simulink model "Sepic_2025b"  (R2025b)
settings: Solver=VariableStepAuto  StartTime=0.0  StopTime=0.02  RelTol=1e-7  AbsTol=1e-7
undefined symbols (not defined in the file): fg_sepic, HPFenable, Ilim_sepic, Ki_sepic, Ku_sepic, R1_sepic, RL_sepic, tau_HPF_sepic, tau_PI_sepic, U2_sepic, w_Amplitude
libraries: fl_lib x14, nesl_utility x12, ee_lib x11, simulink x2, slpidlib x1
settings Model: SimulationMode=accelerator  Creator=Job  LastModifiedBy=jobme
settings SolverCC: AlgebraicLoopSolver=LineSearch  PositivePriorityOrder=on
settings DebuggingCC: UnconnectedInputMsg=warning  UnconnectedOutputMsg=warning  UnconnectedLineMsg=warning
settings HardwareCC: ProdHWDeviceType=AMD->x86-64 (Windows64)
settings ModelReferenceCC: EnableRefExpFcnMdlSchedulingChecks=on
settings SFSimCC: UsePrecompiledLibraries=Avoid  SimTargetLang=C++  GPUAcceleration=on  SimDLTargetLibrary=cudnn
settings RTWCC: GPUComputeCapability=3.5

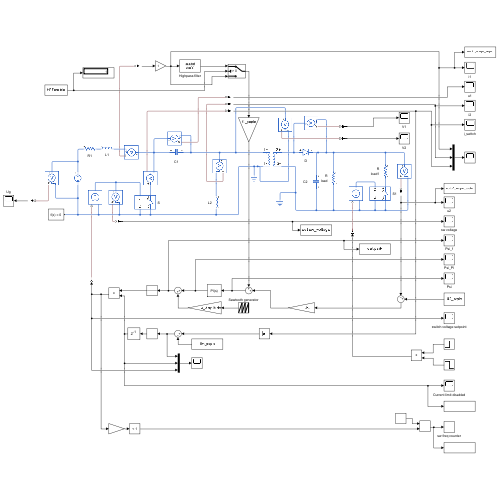
[thumbnail: Simulink's stored preview of the top-level diagram]
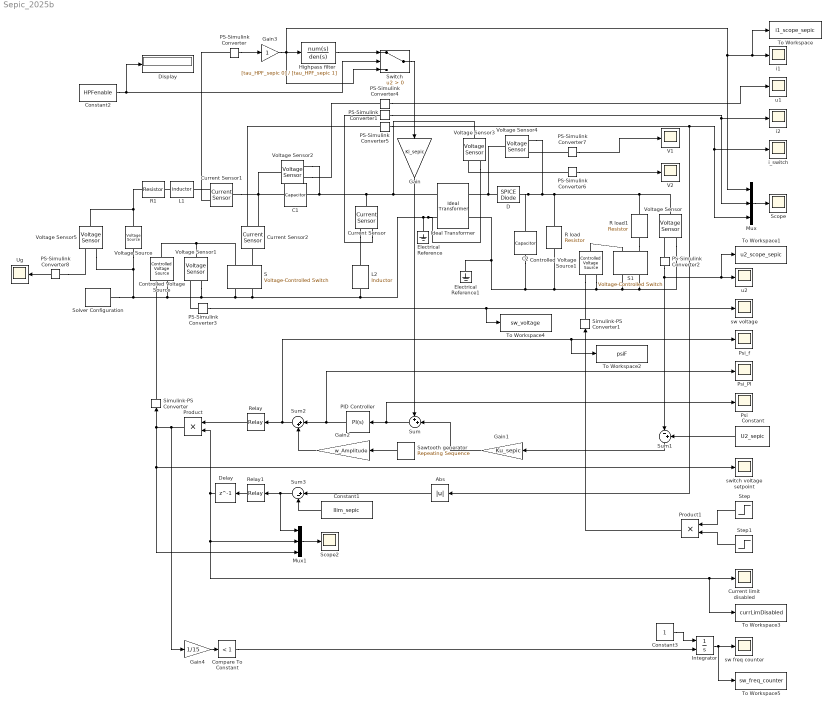
== system Sepic_2025b ==
  Abs : Abs  SaturateOnIntegerOverflow=off
  C1 : ee_lib/Passive/Capacitor  cap_option=ee.enum.passive.capacitor.capOption.const  c=C1_sepic F  Cvec=[1e-05, 1e-06] F  Vvec=[0, 10] V  CV_table_symmetry=1  f_vec=[1, 10] kHz  DFext_vec=[.8, 1.2]  enable_C_tol=0  averaging_period=0 s  C_tol=0  tol_distribution=1  nSigma=4  r=1e-6 Ohm  g=0 1/Ohm  enable_operating_limits=0  operating_limit_action=2  max_working_voltage_range=[-25, 25] V  power_rating=1 W  maxTemperature=85 degC  thermalEnable=false  thermalMass=1 J/K  i_specify=off  i_priority=None  i=0 A  i_nominal_specify=off  i_nominal_value=1  i_nominal_unit=A  v_specify=off  v_priority=None  v=0 V  v_nominal_specify=off  v_nominal_value=1  v_nominal_unit=V  vc_specify=off  vc_priority=High  vc=0 V  vc_nominal_specify=off  vc_nominal_value=1  vc_nominal_unit=V  T_specify=off  T_priority=None  T=298.15 K  T_nominal_specify=off  T_nominal_value=1  T_nominal_unit=K
  C2 : ee_lib/Passive/Capacitor  cap_option=ee.enum.passive.capacitor.capOption.const  c=C2_sepic F  Cvec=[1e-05, 1e-06] F  Vvec=[0, 10] V  CV_table_symmetry=1  f_vec=[1, 10] kHz  DFext_vec=[.8, 1.2]  enable_C_tol=0  averaging_period=0 s  C_tol=0  tol_distribution=1  nSigma=4  r=1e-6 Ohm  g=0 1/Ohm  enable_operating_limits=0  operating_limit_action=2  max_working_voltage_range=[-25, 25] V  power_rating=1 W  maxTemperature=85 degC  thermalEnable=false  thermalMass=1 J/K  i_specify=off  i_priority=None  i=0 A  i_nominal_specify=off  i_nominal_value=1  i_nominal_unit=A  v_specify=off  v_priority=None  v=0 V  v_nominal_specify=off  v_nominal_value=1  v_nominal_unit=V  vc_specify=off  vc_priority=High  vc=0 V  vc_nominal_specify=off  vc_nominal_value=1  vc_nominal_unit=V  T_specify=off  T_priority=None  T=298.15 K  T_nominal_specify=off  T_nominal_value=1  T_nominal_unit=K
  Compare To Constant : simulink/Logic and Bit Operations/Compare To Constant  relop=<  const=1  OutDataTypeStr=boolean
  Constant : Constant  Value=U2_sepic
  Constant1 : Constant  Value=Ilim_sepic
  Constant2 : Constant  Value=HPFenable
  Constant3 : Constant
  Controlled Voltage Source : fl_lib/Electrical/Electrical Sources/Controlled Voltage Source
  Controlled Voltage Source1 : fl_lib/Electrical/Electrical Sources/Controlled Voltage Source
  Current Sensor : fl_lib/Electrical/Electrical Sensors/Current Sensor
  Current Sensor1 : fl_lib/Electrical/Electrical Sensors/Current Sensor
  Current Sensor2 : fl_lib/Electrical/Electrical Sensors/Current Sensor
  Current limit disabled : Scope
      settings: ActiveDisplayYMinimum=-0.125  ActiveDisplayYMaximum=1.125  DataLoggingVariableName=currLimDisabled  DataLoggingSaveFormat=Array
  D : ee_lib/Additional Components/SPICE Semiconductors/SPICE Diode  AREA=1.0 m^2  SCALE=1  IS=1e-14 A/m^2  IKF=Inf A/m^2  ISR=0 A/m^2  N=1  NR=2  M=0.5  VJ=1 V  RS=0.01 m^2*Ohm  C_param=1  CJO=0 F/m^2  FC=0.5  TT=0 s  IC_given=1  V0=0 V  RevBrk=1  BV=Inf V  IBV=1e-3 A/m^2  IBVL=0 A/m^2  NBV=1  NBVL=1  T_param=1  XTI=3.0  EG=1.11 eV  TIKF=0 1/K  TRS1=0 1/K  TRS2=0 1/K^2  TBV1=0 1/K  TBV2=0 1/K^2  TFIXED=300.15 K  TMEAS=300.15 K  TOFFSET=0 K
      settings: InternalSimscapePortConfiguration="{\"Bottom\":[],\"Left\":[{\"id\":\"p\",\"label\":\"+\",\"type\":\"foundation.electrical.electrical\"}],\"Right\":[{\"id\":\"n\",\"label\":\"-\",\"type\":\"foundation.electrical.electrical\"}],\"Top\":[]}"
  Delay : Delay  DelayLength=1
  Display : Display
  Electrical Reference : fl_lib/Electrical/Electrical Elements/Electrical Reference
  Electrical Reference1 : fl_lib/Electrical/Electrical Elements/Electrical Reference
  Gain : Gain  Gain=Ki_sepic
  Gain1 : Gain  Gain=Ku_sepic
  Gain2 : Gain  Gain=w_Amplitude
  Gain3 : Gain
  Gain4 : Gain  Gain=1/15  OutDataTypeStr=uint8
  Highpass filter : TransferFcn  Numerator=[tau_HPF_sepic 0]  Denominator=[tau_HPF_sepic 1]
  Ideal Transformer : fl_lib/Electrical/Electrical Elements/Ideal Transformer  n=n_sepic  i1_specify=off  i1_priority=None  i1=0 A  i1_nominal_specify=off  i1_nominal_value=1  i1_nominal_unit=A  v1_specify=off  v1_priority=None  v1=0 V  v1_nominal_specify=off  v1_nominal_value=1  v1_nominal_unit=V  i2_specify=off  i2_priority=None  i2=0 A  i2_nominal_specify=off  i2_nominal_value=1  i2_nominal_unit=A  v2_specify=off  v2_priority=None  v2=0 V  v2_nominal_specify=off  v2_nominal_value=1  v2_nominal_unit=V
  Integrator : Integrator  ExternalReset=rising
  L1 : ee_lib/Passive/Inductor  l=L1_sepic H  enable_L_tol=0  L_tol=0  tol_distribution=1  nSigma=4  r=0.001 Ohm  g=1e-9 1/Ohm  enable_operating_limits=0  operating_limit_action=2  max_working_current=1 A  power_rating=1 W  i_L_specify=off  i_L_priority=High  i_L=0 A  i_L_nominal_specify=off  i_L_nominal_value=1  i_L_nominal_unit=A
  L2 : ee_lib/Passive/Inductor  l=L2_sepic H  enable_L_tol=0  L_tol=0  tol_distribution=1  nSigma=4  r=0.001 Ohm  g=1e-9 1/Ohm  enable_operating_limits=0  operating_limit_action=2  max_working_current=1 A  power_rating=1 W  i_L_specify=off  i_L_priority=High  i_L=0 A  i_L_nominal_specify=off  i_L_nominal_value=1  i_L_nominal_unit=A
  Mux : Mux  Inputs=3
  Mux1 : Mux  Inputs=3
  PID Controller : slpidlib/PID Controller  Controller=PI  Form=Parallel  TimeDomain=Continuous-time  UseExternalTs=off  SampleTime=-1  IntegratorMethod=Forward Euler  FilterMethod=Forward Euler  ControllerParametersSource=internal  P=1  I=tau_PI_sepic  UseKiTs=off  D=0  UseExternalDerivativeSource=off  N=100  UseFilter=on  TunerSelectOption=Transfer Function Based (PID Tuner App)  InitialConditionSource=internal  InitialConditionForIntegrator=0  InitialConditionForFilter=0  DifferentiatorICPrevScaledInput=0  ExternalReset=none  TrackingMode=off  Kt=1  LimitOutput=off  SatLimitsSource=internal  UpperSaturationLimit=inf  LowerSaturationLimit=-inf  LinearizeAsGain=on  AntiWindupMode=none  Kb=1  LimitIntegrator=off  UpperIntegratorSaturationLimit=inf  LowerIntegratorSaturationLimit=-inf  POutMin=[]  POutMax=[]  IOutMin=[]  IOutMax=[]  DOutMin=[]  DOutMax=[]  NOutMin=[]  NOutMax=[]  SumOutMin=[]  SumOutMax=[]  SaturationOutMin=[]  SaturationOutMax=[]  PParamMin=[]  PParamMax=[]  IParamMin=[]  IParamMax=[]  DParamMin=[]  DParamMax=[]  NParamMin=[]  NParamMax=[]  KbParamMin=[]  KbParamMax=[]  KtParamMin=[]  KtParamMax=[]  KbOutMin=[]  KbOutMax=[]  KtOutMin=[]  KtOutMax=[]  IntegratorOutMin=[]  IntegratorOutMax=[]  FilterOutMin=[]  FilterOutMax=[]  SumI1OutMin=[]  SumI1OutMax=[]  SumI2OutMin=[]  SumI2OutMax=[]  SumI3OutMin=[]  SumI3OutMax=[]  SumI4OutMin=[]  SumI4OutMax=[]  SumDOutMin=[]  SumDOutMax=[]  DifferentiatorOutMin=[]  DifferentiatorOutMax=[]  FilterDiffOutCoefMin=[]  FilterDiffOutCoefMax=[]  ReciprocalOutMin=[]  ReciprocalOutMax=[]  SumDenOutMin=[]  SumDenOutMax=[]  SumNumOutMin=[]  SumNumOutMax=[]  DivideOutMin=[]  DivideOutMax=[]  UdiffTsProdOutMin=[]  UdiffTsProdOutMax=[]  NTsProdOutMin=[]  NTsProdOutMax=[]  UintegralTsProdOutMin=[]  UintegralTsProdOutMax=[]  UngainTsProdOutMin=[]  UngainTsProdOutMax=[]  ClampingZeroOutDataTypeStr=Inherit: Inherit via back propagation  ClampingZeroOutMin=[]  ClampingZeroOutMax=[]  FilterDenConstantOutDataTypeStr=Inherit: Inherit via back propagation  FilterDenConstantOutMin=[]  FilterDenConstantOutMax=[]  PCopyOutDataTypeStr=Inherit: Inherit via back propagation  PCopyOutMin=[]  PCopyOutMax=[]  NCopyOutDataTypeStr=Inherit: Inherit via back propagation  NCopyOutMin=[]  NCopyOutMax=[]  IntegratorContinuousStateAttributes=''  IntegratorStateMustResolveToSignalObject=off  IntegratorRTWStateStorageClass=Auto  FilterContinuousStateAttributes=''  FilterStateMustResolveToSignalObject=off  FilterRTWStateStorageClass=Auto  ParallelPVariant=InternalParameters  IdealPVariant=Disabled  IVariant=InternalParameters  DVariant=Disabled  IntegratorVariant=Continuous  SatVariant=Disabled  AWVariant=Passthrough  PCopyVariant=Disabled  TRVariant=Disabled  FdbkBlocksVariant=Forward  IdealPFdbkVariant=Disabled  SatFdbkVariant=Disabled  DerivativeFilterVariant=Disabled  NVariant=Disabled  NCopyVariant=Disabled_SignalSpec  FilterICVariant=Disabled  IntegratorICVariant=InternalICs  ExternalResetVariant=Disabled  TRSumVariant=Passthrough  SumFdbkVariant=Disabled  SumVariant=Sum_PI  TsampFilterVariant=InternalTs  TsampNgainVariant=Passthrough  TsampIntegralVariant=Disabled_SignalSpec  ExternalSaturationOutDataTypeStr=Inherit: Same as second input  DerivativeSourceVariant=Disabled  PreIntVariant=InternalPreInt
  PS-Simulink Converter{,1..8} (9 alike) : nesl_utility/PS-Simulink Converter  PhysicalDomain=network_engine_domain  SubClassName=ps_output  LeftPortType=input  RightPortType=output  PseudoPeriodic=off  Frequencies=[]  VectorFormat=1-D array  Unit=inherit  AffineConversion=off
  Product : Product
  Product1 : Product
  Psi : Scope
      settings: ActiveDisplayYMinimum=-0.42054  ActiveDisplayYMaximum=0.34086
  Psi_PI : Scope
      settings: ActiveDisplayYMinimum=-0.37093  ActiveDisplayYMaximum=0.39859  DataLoggingVariableName=ScopeData3
  Psi_f : Scope
      settings: ActiveDisplayYMinimum=-5.00943  ActiveDisplayYMaximum=22.85382  DataLoggingDecimation=100  DataLoggingVariableName=psiF  DataLoggingSaveFormat=Array
  R load : ee_lib/Passive/Resistor  R=RL_sepic Ohm  enable_R_tol=0  R_tol=0.001  tol_distribution=1  nSigma=4  enable_operating_limits=0  operating_limit_action=2  power_rating=1 W  max_working_voltage=100 V  noise_mode=0  Tdevice=25 degC  sample_time=1e-3 s  repeatability=1  user_seed=0  auto_seed=1005501763  power_derating_T1=70 degC  power_derating_T2=155 degC  operating_temperature_range_vec=[-50, 150] degC  alpha=3.93e-3 1/K  Tmeas=25 degC  thermal_mass=100 J/K  temperature_specify=off  temperature_priority=High  temperature=298.15 K  temperature_nominal_specify=off  temperature_nominal_value=1  temperature_nominal_unit=K
  R load1 : ee_lib/Passive/Resistor  R=22.222 Ohm  enable_R_tol=0  R_tol=0.001  tol_distribution=1  nSigma=4  enable_operating_limits=0  operating_limit_action=2  power_rating=1 W  max_working_voltage=100 V  noise_mode=0  Tdevice=25 degC  sample_time=1e-3 s  repeatability=1  user_seed=0  auto_seed=2350272805  power_derating_T1=70 degC  power_derating_T2=155 degC  operating_temperature_range_vec=[-50, 150] degC  alpha=3.93e-3 1/K  Tmeas=25 degC  thermal_mass=100 J/K  temperature_specify=off  temperature_priority=High  temperature=298.15 K  temperature_nominal_specify=off  temperature_nominal_value=1  temperature_nominal_unit=K
  R1 : ee_lib/Passive/Resistor  R=R1_sepic Ohm  enable_R_tol=0  R_tol=0.1  tol_distribution=1  nSigma=4  enable_operating_limits=0  operating_limit_action=2  power_rating=1 W  max_working_voltage=100 V  noise_mode=0  Tdevice=25 degC  sample_time=1e-3 s  repeatability=1  user_seed=0  auto_seed=551673987  power_derating_T1=70 degC  power_derating_T2=155 degC  operating_temperature_range_vec=[-50, 150] degC  alpha=3.93e-3 1/K  Tmeas=25 degC  thermal_mass=100 J/K  temperature_specify=off  temperature_priority=High  temperature=298.15 K  temperature_nominal_specify=off  temperature_nominal_value=1  temperature_nominal_unit=K
  Relay : Relay  OnSwitchValue=0.15  OffSwitchValue=-0.15  OnOutputValue=15
  Relay1 : Relay  OnSwitchValue=0  OffSwitchValue=-0.5  OnOutputValue=0  OffOutputValue=1
  S : ee_lib/Additional Components/SPICE Passives/Voltage-Controlled Switch  SWITCH_model=ee.enum.switches.switchModelVoltage.transition  VON=1 V  VOFF=0 V  VT=1 V  VH=0 V  RON=0.0001 Ohm  ROFF_res=1e6 Ohm  Roff_gmin=ee.enum.switches.offResistance.no  ROFF=10e6 Ohm  TD=0 s
      settings: InternalSimscapePortConfiguration="{\"Bottom\":[],\"Left\":[{\"id\":\"p1\",\"label\":\"1+\",\"type\":\"foundation.electrical.electrical\"},{\"id\":\"p2\",\"label\":\"2+\",\"type\":\"foundation.electrical.electrical\"}],\"Right\":[{\"id\":\"n1\",\"label\":\"1-\",\"type\":\"foundation.electrical.electrical\"},{\"id\":\"n2\",\"label\":\"2-\",\"type\":\"foundation.electrical.electrical\"}],\"Top\":[]}"
  S1 : ee_lib/Additional Components/SPICE Passives/Voltage-Controlled Switch  SWITCH_model=ee.enum.switches.switchModelVoltage.transition  VON=1 V  VOFF=0 V  VT=1 V  VH=0 V  RON=0.0001 Ohm  ROFF_res=1e6 Ohm  Roff_gmin=ee.enum.switches.offResistance.no  ROFF=10e6 Ohm  TD=0 s
      settings: InternalSimscapePortConfiguration="{\"Bottom\":[],\"Left\":[{\"id\":\"p1\",\"label\":\"1+\",\"type\":\"foundation.electrical.electrical\"},{\"id\":\"p2\",\"label\":\"2+\",\"type\":\"foundation.electrical.electrical\"}],\"Right\":[{\"id\":\"n1\",\"label\":\"1-\",\"type\":\"foundation.electrical.electrical\"},{\"id\":\"n2\",\"label\":\"2-\",\"type\":\"foundation.electrical.electrical\"}],\"Top\":[]}"
  Sawtooth generator : simulink/Sources/Repeating Sequence  rep_seq_t=[0 1/fg_sepic]  rep_seq_y=[0 1]
  Scope : Scope
      settings: ActiveDisplayYMinimum=-237.72024375100756  ActiveDisplayYMaximum=2015.3547129226815
  Scope2 : Scope
      settings: ActiveDisplayYMinimum=-4.5625  ActiveDisplayYMaximum=6.0625  DataLoggingVariableName=ScopeData5
  Simulink-PS Converter : nesl_utility/Simulink-PS Converter  PhysicalDomain=network_engine_domain  SubClassName=ps_input  LeftPortType=input  RightPortType=output  PseudoPeriodic=off  Frequencies=[]  NoiseDistribution=none  NoiseParameters=[]  Unit=1  AffineConversion=off  FilteringAndDerivatives=provide  SimscapeFilterOrder=1  InputFilterTimeConstant=0.001  UdotUserProvided=0
  Simulink-PS Converter1 : nesl_utility/Simulink-PS Converter  PhysicalDomain=network_engine_domain  SubClassName=ps_input  LeftPortType=input  RightPortType=output  PseudoPeriodic=off  Frequencies=[]  NoiseDistribution=none  NoiseParameters=[]  Unit=1  AffineConversion=off  FilteringAndDerivatives=provide  SimscapeFilterOrder=1  InputFilterTimeConstant=0.001  UdotUserProvided=0
  Solver Configuration : nesl_utility/Solver Configuration  PhysicalDomain=network_engine_domain  SubClassName=solver  LeftPortType=input  RightPortType=generic  Tones=[]  Harmonics=[]  SimulateNoise=off  Profile=off  UseLocalSampling=off  EnableSwitchedLinearOptims=on  FrequencyDomain=off  UseCCode=off  RelTol=0.001  AbsTol=1e-06  MinStep=1e-09  ToWorkspace=off  RevertToSquareIcSolve=off  NumHomotopyIterations=100  PhasorMode=off  PhasorModeNumHarmonics=1  ConsistencySolver=NEWTON_FTOL  IndexReductionMethod=DerivativeReplacement  DoDC=on  ResidualTolerance=1e-09  ConsistencyTolSource=GLOBAL  ConsistencyAbsTol=0.001  ConsistencyRelTol=0.001  ConsistencyTolFactor=0.001  UseLocalSolver=off  LocalSolverChoice=NE_PARTITIONING_ADVANCER  ResolveIndetEquations=on  FunctionEvalNumThread=1  LocalSolverSampleTime=1e-9  DoFixedCost=off  MaxNonlinIter=3  MaxModeIter=2  ComputeImpulses=off  ImpulseIterations=2  LinearAlgebra=auto  LinearAlgebraNumThread=0  EquationFormulation=NE_TIME_EF  DelaysMemoryBudget=1024  AutomaticFiltering=off  FilteringTimeConstant=0.001  PartitionStorageMethod=AS_NEEDED  PartitionMemoryBudget=1024  PartitionMethod=ROBUST  MultibodyUseLocalSolver=off  MultibodyLocalSolverChoice=ODE1  MultibodyLocalSolverSampleTime=0.001
  Step : Step  Time=0.01  After=5  SampleTime=0
  Step1 : Step  Time=0.015  Before=1  After=0  SampleTime=0
  Sum : Sum  Inputs=++|
  Sum1 : Sum  Inputs=|-+
  Sum2 : Sum  Inputs=|++
  Sum3 : Sum  Inputs=|+-
  Switch : Switch  Criteria=u2 > Threshold  SaturateOnIntegerOverflow=off  InputSameDT=off
  To Workspace : ToWorkspace  VariableName=i1_scope_sepic  SaveFormat=Timeseries  SampleTime=-1
  To Workspace1 : ToWorkspace  VariableName=u2_scope_sepic  SaveFormat=Timeseries  SampleTime=-1
  To Workspace2 : ToWorkspace  VariableName=psiF  SaveFormat=Timeseries  SampleTime=-1
  To Workspace3 : ToWorkspace  VariableName=currLimDisabled  SaveFormat=Timeseries  SampleTime=-1
  To Workspace4 : ToWorkspace  VariableName=sw_voltage  SaveFormat=Timeseries  SampleTime=-1
  To Workspace5 : ToWorkspace  VariableName=sw_freq_counter  SaveFormat=Timeseries  SampleTime=-1
  Ug : Scope
      settings: ActiveDisplayYMinimum=-10.79879  ActiveDisplayYMaximum=38.46445
  V1 : Scope
      settings: ActiveDisplayYMinimum=-52.30801  ActiveDisplayYMaximum=6.89341
  V2 : Scope
      settings: ActiveDisplayYMinimum=-49.74927  ActiveDisplayYMaximum=45.41628  DataLoggingVariableName=ScopeData2
  Voltage Sensor{,1..5} (6 alike) : fl_lib/Electrical/Electrical Sensors/Voltage Sensor
  Voltage Source : ee_lib/Sources/Voltage Source  dc_voltage=Ug_sepic V  ac_voltage=4.5 V  ac_shift=0 rad  ac_frequency=100 Hz  noise_mode=0  PSD=0 V^2/Hz  sample_time=1e-3 s  repeatability=1  user_seed=0  auto_seed=2816384857  i_specify=off  i_priority=None  i=0 A  i_nominal_specify=off  i_nominal_value=1  i_nominal_unit=A  v_specify=off  v_priority=None  v=0 V  v_nominal_specify=off  v_nominal_value=1  v_nominal_unit=V
  i1 : Scope
      settings: ActiveDisplayYMinimum=-14.203562358386067  ActiveDisplayYMaximum=9.8085065736953059  DataLoggingDecimation=100  DataLoggingVariableName=i1_scope_sepic  DataLoggingSaveFormat=Array
  i2 : Scope
      settings: ActiveDisplayYMinimum=-3.87101  ActiveDisplayYMaximum=2.72088
  i_switch : Scope
      settings: ActiveDisplayYMinimum=-6.60412  ActiveDisplayYMaximum=0.73379  DataLoggingVariableName=ScopeData2
  sw freq counter : Scope
      settings: ActiveDisplayYMinimum=-0.00025  ActiveDisplayYMaximum=0.00223  DataLoggingVariableName=ScopeData3
  sw voltage : Scope
      settings: ActiveDisplayYMinimum=-1.875  ActiveDisplayYMaximum=16.875  DataLoggingVariableName=sw_voltage  DataLoggingSaveFormat=Array
  switch voltage setpoint : Scope
      settings: ActiveDisplayYMinimum=-1.875  ActiveDisplayYMaximum=16.875  DataLoggingVariableName=ScopeData3
  u1 : Scope
      settings: ActiveDisplayYMinimum=-10.79879  ActiveDisplayYMaximum=38.46445
  u2 : Scope
      settings: ActiveDisplayYMinimum=-3.0218010471894776  ActiveDisplayYMaximum=27.196209424650924  DataLoggingDecimation=100  DataLoggingVariableName=u2_scope_sepic  DataLoggingSaveFormat=Array
  wires:
  PS-Simulink Converter1/1 -> Mux/2, i2/1
  PS-Simulink Converter3/1 -> sw voltage/1, To Workspace4/1
  Gain3/1 -> Highpass filter/1, Switch/3, Mux/1, To Workspace/1, i1/1
  PS-Simulink Converter/1 -> Gain3/1
  PS-Simulink Converter2/1 -> Sum1/1, To Workspace1/1, u2/1
  Gain1/1 -> Sum/2
  Gain/1 -> Sum/1
  Sum/1 -> Psi/1, PID Controller/1
  Sum1/1 -> Gain1/1
  Constant/1 -> Sum1/2
  PS-Simulink Converter4/1 -> u1/1
  PS-Simulink Converter5/1 -> Mux/3, i_switch/1, Abs/1
  Sawtooth generator/1 -> Gain2/1
  Sum2/1 -> Relay/1, Psi_f/1, To Workspace2/1
  Gain2/1 -> Sum2/2
  PS-Simulink Converter7/1 -> V1/1
  PS-Simulink Converter6/1 -> V2/1
  Product/1 -> Simulink-PS Converter/1, Mux1/3, switch voltage setpoint/1, Gain4/1
  Constant1/1 -> Sum3/2
  Abs/1 -> Sum3/1
  Relay/1 -> Product/1
  Sum3/1 -> Mux1/1, Relay1/1
  Relay1/1 -> Delay/1
  Delay/1 -> Product/2, To Workspace3/1, Current limit disabled/1, Mux1/2
  Mux1/1 -> Scope2/1
  Mux/1 -> Scope/1
  Product1/1 -> Simulink-PS Converter1/1
  Step/1 -> Product1/1
  Step1/1 -> Product1/2
  PID Controller/1 -> Psi_PI/1, Sum2/1
  Highpass filter/1 -> Switch/1
  Switch/1 -> Gain/1
  Constant2/1 -> Display/1, Switch/2
  PS-Simulink Converter8/1 -> Ug/1
  Gain4/1 -> Compare To Constant/1
  Constant3/1 -> Integrator/1
  Compare To Constant/1 -> Integrator/2
  Integrator/1 -> To Workspace5/1, sw freq counter/1
  connections:
  D/RConn1 -- Voltage Sensor4/RConn2 -- R load1/LConn1 -- Voltage Sensor/LConn1 -- R load/LConn1 -- C2/LConn1
  Voltage Sensor1/LConn1 -- Controlled Voltage Source/LConn1 -- S/LConn1
  S1/RConn1 -- S1/RConn2 -- Voltage Sensor/RConn2 -- Controlled Voltage Source1/RConn2 -- R load/RConn1 -- C2/RConn1 -- Ideal Transformer/RConn2 -- Electrical Reference1/LConn1
  C1/LConn1 -- Current Sensor1/LConn1 -- Voltage Sensor2/LConn1 -- Current Sensor2/RConn2
  Current Sensor/RConn1 -- PS-Simulink Converter1/LConn1
  Current Sensor1/RConn1 -- PS-Simulink Converter/LConn1
  PS-Simulink Converter3/LConn1 -- Voltage Sensor1/RConn1
  Voltage Source/LConn1 -- Voltage Sensor5/LConn1 -- R1/LConn1
  PS-Simulink Converter2/LConn1 -- Voltage Sensor/RConn1
  L1/LConn1 -- R1/RConn1
  Ideal Transformer/LConn1 -- Voltage Sensor3/LConn1 -- Current Sensor/LConn1 -- Voltage Sensor2/RConn2 -- C1/RConn1
  L2/RConn1 -- Electrical Reference/LConn1 -- Voltage Sensor3/RConn2 -- Ideal Transformer/LConn2 -- Voltage Sensor1/RConn2 -- Voltage Sensor5/RConn2 -- Voltage Source/RConn1 -- Solver Configuration/RConn1 -- Controlled Voltage Source/RConn2 -- S/RConn1 -- S/RConn2
  D/LConn1 -- Ideal Transformer/RConn1 -- Voltage Sensor4/LConn1
  Simulink-PS Converter/RConn1 -- Controlled Voltage Source/RConn1
  L1/RConn1 -- Current Sensor1/RConn2
  Current Sensor/RConn2 -- L2/LConn1
  Voltage Sensor2/RConn1 -- PS-Simulink Converter4/LConn1
  S/LConn2 -- Current Sensor2/LConn1
  Current Sensor2/RConn1 -- PS-Simulink Converter5/LConn1
  PS-Simulink Converter6/LConn1 -- Voltage Sensor3/RConn1
  PS-Simulink Converter7/LConn1 -- Voltage Sensor4/RConn1
  R load1/RConn1 -- S1/LConn2
  Controlled Voltage Source1/LConn1 -- S1/LConn1
  Controlled Voltage Source1/RConn1 -- Simulink-PS Converter1/RConn1
  PS-Simulink Converter8/LConn1 -- Voltage Sensor5/RConn1
